simulink model "Q12_Sim"  (R2023b)
settings: Solver=VariableStepAuto  StartTime=0.0  StopTime=10.0  RelTol=1e-3
values from neighbouring files (symbols this model uses):
  den = cell2mat(den)    [Quest_12.m]
  num = cell2mat(num)    [Quest_12.m]
settings Model: Creator=GEPAE1  LastModifiedBy=Lucas
settings SolverCC: AlgebraicLoopSolver=TrustRegion
settings DebuggingCC: UnconnectedInputMsg=warning  UnconnectedOutputMsg=warning  UnconnectedLineMsg=warning
settings ModelReferenceCC: EnableRefExpFcnMdlSchedulingChecks=on

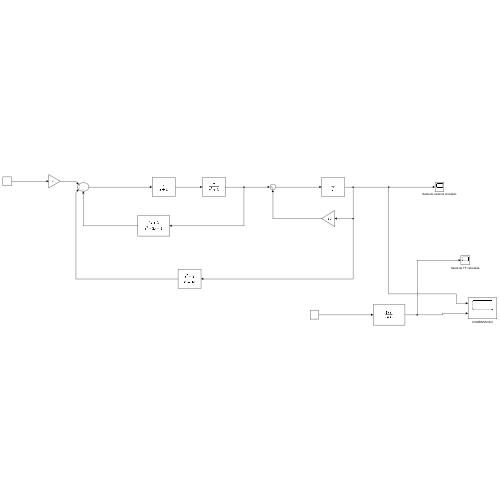
[thumbnail: Simulink's stored preview of the top-level diagram]
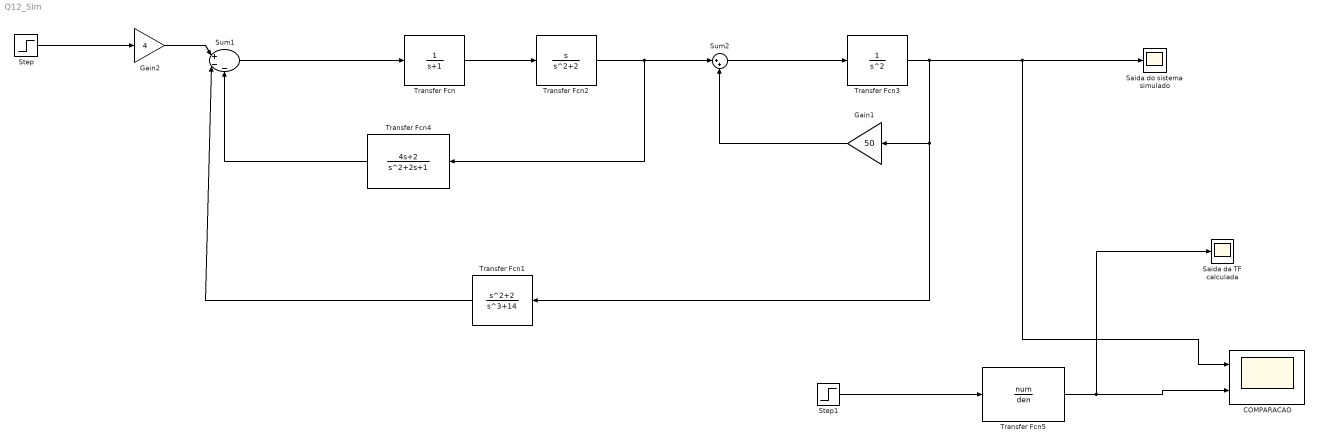
== system Q12_Sim ==
  COMPARACAO : Scope  NumInputPorts=2
  Gain1 : Gain  Gain=50
  Gain2 : Gain  Gain=4
  Saida da TF calculada : Scope
  Saida do sistema simulado : Scope
  Step : Step  Time=0  SampleTime=0
  Step1 : Step  Time=0  SampleTime=0
  Sum1 : Sum  Inputs=|+--
  Sum2 : Sum  Inputs=|++
  Transfer Fcn : TransferFcn  Denominator=[1 1]
  Transfer Fcn1 : TransferFcn  Numerator=[1 0 2]  Denominator=[1 0 0 14]
  Transfer Fcn2 : TransferFcn  Numerator=[1 0]  Denominator=[1 0 2]
  Transfer Fcn3 : TransferFcn  Denominator=[1 0 0]
  Transfer Fcn4 : TransferFcn  Numerator=[4 2]
  Transfer Fcn5 : TransferFcn  Numerator=num  Denominator=den
  wires:
  Transfer Fcn/1 -> Transfer Fcn2/1
  Sum1/1 -> Transfer Fcn/1
  Transfer Fcn2/1 -> Sum2/1, Transfer Fcn4/1
  Sum2/1 -> Transfer Fcn3/1
  Gain1/1 -> Sum2/2
  Transfer Fcn1/1 -> Sum1/2
  Transfer Fcn4/1 -> Sum1/3
  Gain2/1 -> Sum1/1
  Step/1 -> Gain2/1
  Transfer Fcn5/1 -> Saida da TF calculada/1, COMPARACAO/2
  Step1/1 -> Transfer Fcn5/1
  Transfer Fcn3/1 -> COMPARACAO/1, Saida do sistema simulado/1, Transfer Fcn1/1, Gain1/1
